simulink model "la06"  (R2017a)
settings: Solver=VariableStepAuto  StartTime=0.0  StopTime=inf  RelTol=1e-3
libraries: dspvision x2, dspsnks4 x1
settings Model: Creator=HP  LastModifiedBy=HP

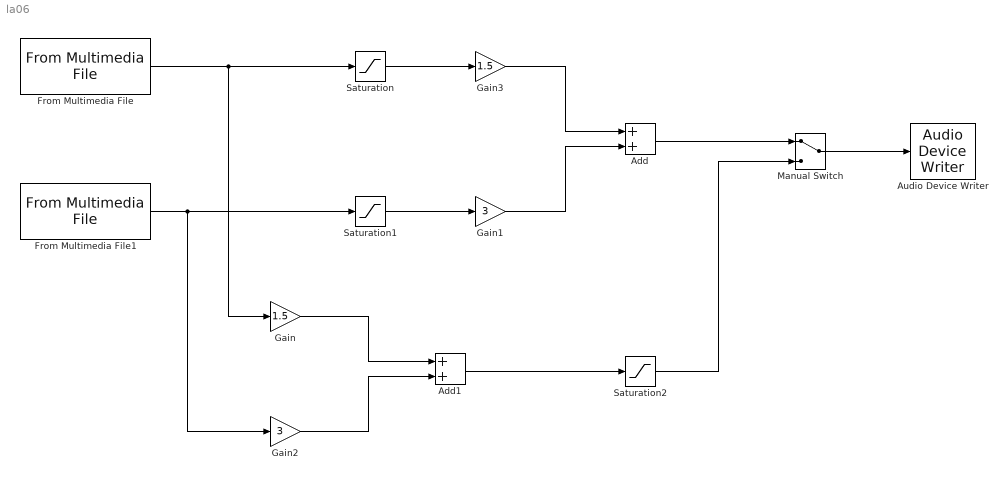
== system la06 ==
  Add : Sum
  Add1 : Sum
  Audio Device Writer : dspsnks4/Audio Device Writer  Driver=DirectSound  Device=Default  InheritSampleRate=on  SampleRate=44100  BitDepth=16-bit integer  BufferSize=4096  NumBuffers=10  DefaultOutputChannelMapping=on  OutputChannelMapping=1:2  OutputNumUnderrunSamples=off  DriverIdx=1  DeviceWarnFlag=''
  From Multimedia File : dspvision/From Multimedia File  inputFilename="C:\\Users\\HP\\Google Drive\\Year 2\\Semester 2\\SIGNALS AND SYSTEMS  EC2112 [2021JUL]\\signals-and-systems\\lab 2\\VoiceOnly.wav"  loop=on  numPlays=inf  outputStreams=Audio only  videoDataType=single  audioDataType=double  inheritSampleTime=on  userDefinedSampleTime=1/30  noAudioOutput=off  isIntensityVideo=off  fourcc=RGB  colorVideoFormat=Separate color signals  outputEOF=off  dataOrg=Column-major  audioFrameSize=1024  computeAudioFrameSize=off  outSamplingMode=Sample based
      settings: SourceProductBaseCode=VP
  From Multimedia File1 : dspvision/From Multimedia File  inputFilename="C:\\Users\\HP\\Google Drive\\Year 2\\Semester 2\\SIGNALS AND SYSTEMS  EC2112 [2021JUL]\\signals-and-systems\\lab 2\\MusicOnly.wav"  loop=on  numPlays=inf  outputStreams=Audio only  videoDataType=single  audioDataType=double  inheritSampleTime=on  userDefinedSampleTime=1/30  noAudioOutput=off  isIntensityVideo=off  fourcc=RGB  colorVideoFormat=Separate color signals  outputEOF=off  dataOrg=Column-major  audioFrameSize=1024  computeAudioFrameSize=off  outSamplingMode=Sample based
      settings: SourceProductBaseCode=VP
  Gain : Gain  Gain=1.5
  Gain1 : Gain  Gain=3
  Gain2 : Gain  Gain=3
  Gain3 : Gain  Gain=1.5
  Manual Switch : ManualSwitch
  Saturation : Saturate  UpperLimit=10  LowerLimit=-10
  Saturation1 : Saturate  UpperLimit=10  LowerLimit=-10
  Saturation2 : Saturate  UpperLimit=10  LowerLimit=-10
  wires:
  Add/1 -> Manual Switch/1
  Saturation2/1 -> Manual Switch/2
  Gain3/1 -> Add/1
  Saturation1/1 -> Gain1/1
  From Multimedia File/1 -> Gain/1, Saturation/1
  From Multimedia File1/1 -> Gain2/1, Saturation1/1
  Gain1/1 -> Add/2
  Add1/1 -> Saturation2/1
  Gain/1 -> Add1/1
  Manual Switch/1 -> Audio Device Writer/1
  Gain2/1 -> Add1/2
  Saturation/1 -> Gain3/1
